simulink model "test_loadcase_moduleAssy_harness"  (R2026a)
settings: Solver=VariableStepAuto  StopTime=2000  AbsTol=1e-3
libraries: cooling_system_components x9, fl_lib x3, simulink x2, nesl_utility x2, pack_5p48s8p_detailled_Thr_library x1, pack_5p48s8p_1g10g1_Thr_library x1, pack_5p48s8p_1g10g1_5g1g5_Thr_library x1, pack_5p48s8p_Thr_library x1
Description:
  | Copyright 2023-2026 The MathWorks, Inc.
settings Model: Creator=smiller  LastModifiedBy=smiller
settings DebuggingCC: SymbolicDimsDataTypeCodeGenerationDiagnostic=none
settings SimscapeCC: SimscapeNominalValues="[{\"value\":\"1\",\"unit\":\"A\"},{\"value\":\"1\",\"unit\":\"bar\"},{\"value\":\"1\",\"unit\":\"cm^2\"},{\"value\":\"1\",\"unit\":\"cm^3/s\"},{\"value\":\"1\",\"unit\":\"kJ/kg\"},{\"value\":\"1\",\"unit\":\"kW\"},{\"value\":\"1\",\"unit\":\"l\"},{\"value\":\"1\",\"unit\":\"N\"},{\"value\":\"1\",\"unit\":\"N*m\"},{\"value\":\"1\",\"unit\":\"V\"}]"  SimscapeLogSimulationStatistics=on  SimscapeLogName=simlog_test_loadcase_module

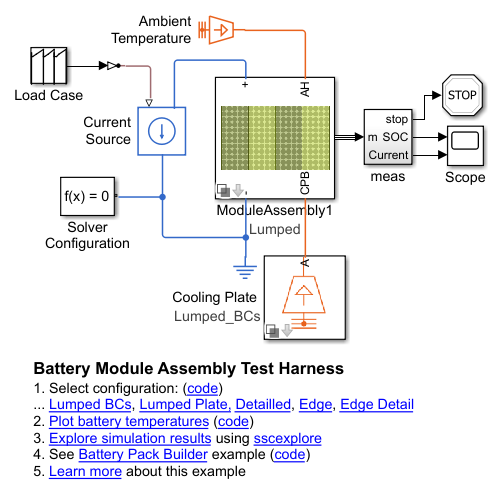
[thumbnail: Simulink's stored preview of the top-level diagram]
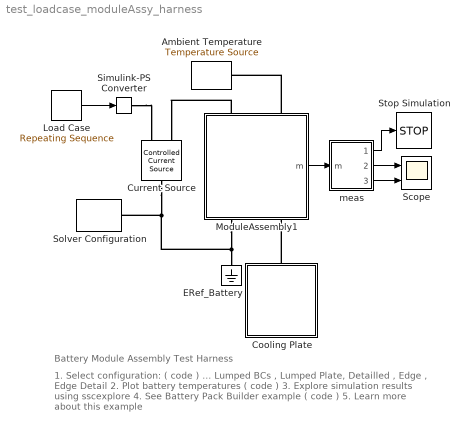
== system test_loadcase_moduleAssy_harness ==
  note: 1. Select configuration: ( code )
      | ... Lumped BCs , Lumped Plate, Detailled , Edge , Edge Detail
      | 2. Plot battery temperatures ( code )
      | 3. Explore simulation results using sscexplore
      | 4. See Battery Pack Builder example ( code )
      | 5. Learn more about this example
  note: Battery Module Assembly Test Harness
  Ambient Temperature : fl_lib/Thermal/Thermal Sources/Temperature Source  temperature=298 K
  Cooling Plate : Subsystem  Variant=on  VariantControlMode=label  VariantControl=Lumped_BCs  LabelModeActiveChoice=Lumped_BCs
      settings: AttributesFormatString=%<LabelModeActiveChoice>
  Current Source : fl_lib/Electrical/Electrical Sources/Controlled Current Source
  ERef_Battery : fl_lib/Electrical/Electrical Elements/Electrical Reference
  Load Case : simulink/Sources/Repeating Sequence  rep_seq_t="[0 1   2    32  33 300 800 2000]"  rep_seq_y=[0 0 450 450 400 400 440 510]/8
  ModuleAssembly1 : Subsystem  Variant=on  VariantControlMode=label  VariantControl=Choice  LabelModeActiveChoice=Lumped
      settings: AttributesFormatString=%<LabelModeActiveChoice>  PortSchema="{\"entries\":[{\"content\":{\"sides\":[{\"content\":{\"connectorIds\":[\"LConn1\",\"LConn2\"]},\"type\":\"ConnectorPlacement.EquallySpacedRectSide\",\"uuid\":\"bc91a472-35c0-4041-89a6-b649b08794f0\"},{\"content\":{\"connectorIds\":[\"RConn1\",\"RConn2\"],\"side\":\"RIGHT\"},\"type\":\"ConnectorPlacement.EquallySpacedRectSide\",\"uuid\":\"4a390b53-12a2-4d2f-9537-abc76db307f8\"},{\"content\":{\"connectorIds\":[],\"side\":\"TOP\"},\"type\":\"ConnectorPlacement.EquallySpacedRectSide\",\"uuid\":\"1a7ed896-4ada-4d88-995c-c24bd39ee86b\"},{\"content\":{\"connectorIds\":[\"Out1\"],\"side\":\"BOTTOM\"},\"type\":\"ConnectorPlacement.EquallySpacedRectSide\",\"uuid\":\"e36c911b-adc9-44cf-bfab-32777b2ec35c\"}]},\"type\":\"ConnectorPlacement.EquallySpacedConnector\",\"uuid\":\"4e67d65b-f12d-4d00-91b0-7eadb0a42625\"}],\"packageUris\":[\"http://schema.mathworks.com/mf0/Connector/R2020b\"],\"version\":\"1.0\"}"
  Scope : Scope  NumInputPorts=2
      settings: Title=Battery SOC  ActiveDisplayYMinimum=0.2125000000000116  ActiveDisplayYMaximum=1.0874999999999988
  Simulink-PS Converter : nesl_utility/Simulink-PS Converter  PhysicalDomain=network_engine_domain  SubClassName=ps_input  LeftPortType=input  RightPortType=output  PseudoPeriodic=off  Frequencies=[]  NoiseDistribution=none  NoiseParameters=[]  Unit=1  AffineConversion=off  FilteringAndDerivatives=filter  SimscapeFilterOrder=1  InputFilterTimeConstant=0.01  UdotUserProvided=0
  Solver Configuration : nesl_utility/Solver Configuration  PhysicalDomain=network_engine_domain  SubClassName=solver  LeftPortType=input  RightPortType=generic  Tones=[]  Harmonics=[]  SimulateNoise=off  Profile=off  UseLocalSampling=off  EnableSwitchedLinearOptims=on  FrequencyDomain=off  UseCCode=off  RelTol=0.001  AbsTol=1e-06  MinStep=1e-09  ToWorkspace=off  RevertToSquareIcSolve=off  NumHomotopyIterations=100  PhasorMode=off  PhasorModeNumHarmonics=1  ConsistencySolver=NEWTON_XTOL_AFTER_FTOL  CanonicalOrdering=UNORDERED  OptimizeIntermediates=UNOPTIMIZED  IndexReductionMethod=None  DoDC=off  ResidualTolerance=1e-09  ConsistencyTolSource=GLOBAL  ConsistencyAbsTol=0.001  ConsistencyRelTol=0.001  ConsistencyTolFactor=0.001  UseLocalSolver=off  LocalSolverChoice=NE_BACKWARD_EULER_ADVANCER  ResolveIndetEquations=on  FunctionEvalNumThread=1  LocalSolverSampleTime=0.001  DoFixedCost=off  MaxNonlinIter=3  MaxModeIter=2  ComputeImpulses=off  ImpulseIterations=2  LinearAlgebra=auto  LinearAlgebraNumThread=0  EquationFormulation=NE_TIME_EF  DelaysMemoryBudget=1024  AutomaticFiltering=on  FilteringTimeConstant=0.001  PartitionStorageMethod=AS_NEEDED  PartitionMemoryBudget=1024  PartitionMethod=ROBUST  MultibodyUseLocalSolver=off  MultibodyLocalSolverChoice=ODE1  MultibodyLocalSolverSampleTime=0.001
  Stop Simulation : Stop
  meas : Subsystem
  wires:
  Load Case/1 -> Simulink-PS Converter/1
  ModuleAssembly1/1(m) -> meas/1(m)
  meas/1(stop) -> Stop Simulation/1
  meas/2(SOC) -> Scope/1
  meas/3(Current) -> Scope/2
  connections:
  Solver Configuration/RConn1 -- ModuleAssembly1/RConn1 -- ERef_Battery/LConn1 -- Current Source/LConn1
  Simulink-PS Converter/RConn1 -- Current Source/RConn1
  ModuleAssembly1/LConn1 -- Current Source/RConn2
  ModuleAssembly1/LConn2 -- Ambient Temperature/LConn1
  Cooling Plate/LConn1 -- ModuleAssembly1/RConn2

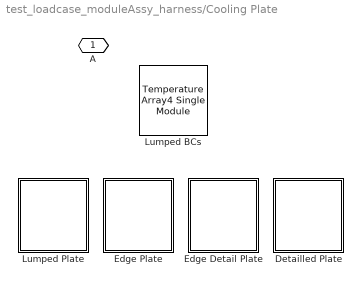
== system test_loadcase_moduleAssy_harness/Cooling Plate ==
  Detailled Plate : Subsystem  VariantControl=Detailled_Plate
      mask Display: image('ssc_airvtol_cooling_plate_IMAGE.png');
  Edge Plate : Subsystem  VariantControl=Edge_Plate
      mask Display: image('ssc_airvtol_cooling_plate_IMAGE.png');
  Edge Detail Plate : Subsystem  VariantControl=Edge_Detail_Plate
      mask Display: image('ssc_airvtol_cooling_plate_IMAGE.png');
  Lumped BCs : cooling_system_components/Temperature Array4 Single Module  VariantControl=Lumped_BCs  t_in=23  t_out=26
  Lumped Plate : Subsystem  VariantControl=Lumped_Plate
      mask Display: image('ssc_airvtol_cooling_plate_IMAGE.png');
  A : PMIOPort  Side=Left

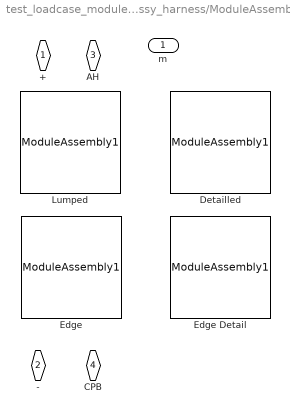
== system test_loadcase_moduleAssy_harness/ModuleAssembly1 ==
  Detailled : pack_5p48s8p_detailled_Thr_library/ModuleAssembly1  VariantControl=Detailled  Cell=ModuleType1_det  Targets=targets_5p48s8p_detailled_thr.ModuleAssembly1  BatteryObj=batt_5p12s_detailled_thr
  Edge : pack_5p48s8p_1g10g1_Thr_library/ModuleAssembly1  VariantControl=Edge  Cell=ModuleType1  Targets=targets_5p48s8p_1g10g1_thr.ModuleAssembly1  BatteryObj=batt_5p48s_1g10g1_thr
  Edge Detail : pack_5p48s8p_1g10g1_5g1g5_Thr_library/ModuleAssembly1  VariantControl=Edge_Detail  Cell=ModuleType1  Targets=targets_5p48s8p_1g10g1_5g1g5_thr.ModuleAssembly1  BatteryObj=batt_5p48s_1g10g1_5g1g5_thr
  Lumped : pack_5p48s8p_Thr_library/ModuleAssembly1  VariantControl=Lumped  Cell=ModuleType1  Targets=targets_5p48s8p_thr.ModuleAssembly1  BatteryObj=batt_5p48s_thr
  + : PMIOPort  Side=Left
  - : PMIOPort  Port=2  Side=Right
  AH : PMIOPort  Port=3  Side=Left
  CPB : PMIOPort  Port=4  Side=Right
  m : Outport

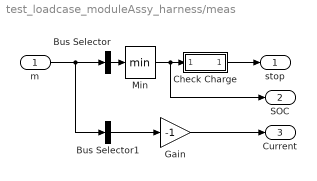
== system test_loadcase_moduleAssy_harness/meas ==
  m : Inport
  Bus Selector : BusSelector  OutputSignals=socC.M1  OutputAsBus=on
  Bus Selector1 : BusSelector  OutputSignals=i.M1  OutputAsBus=on
  Check Charge : Subsystem  mask{q_battery_limit=0.3}
      mask prompts: q_battery_limit "Battery charge lower limit (A*hr)"
  Gain : Gain  Gain=-1
  Min : MinMax
  stop : Outport
  SOC : Outport  Port=2
  Current : Outport  Port=3
  wires:
  Min/1 -> SOC/1, Check Charge/1(In1)
  m/1 -> Bus Selector1/1, Bus Selector/1
  Bus Selector1/1 -> Gain/1
  Bus Selector/1 -> Min/1
  Check Charge/1(stop) -> stop/1
  Gain/1 -> Current/1

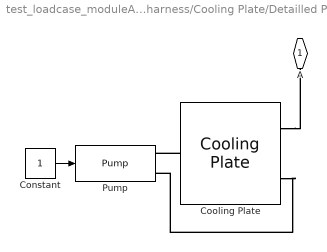
== system test_loadcase_moduleAssy_harness/Cooling Plate/Detailled Plate ==
  Constant : Constant
  Cooling Plate : cooling_system_components/Cooling Plate  plate=plate_5p48s_detailled_thr
  Pump : cooling_system_components/Pump  num_plates=1
  A : PMIOPort  Side=Left
  wires:
  Constant/1 -> Pump/1
  connections:
  Cooling Plate/LConn2 -- Pump/RConn2
  Cooling Plate/RConn1 -- Pump/RConn1
  Cooling Plate/LConn1 -- A/RConn1

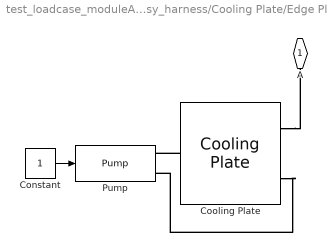
== system test_loadcase_moduleAssy_harness/Cooling Plate/Edge Plate ==
  Constant : Constant
  Cooling Plate : cooling_system_components/Cooling Plate  plate=plate_5p48s_1g10g1_thr
  Pump : cooling_system_components/Pump  num_plates=1
  A : PMIOPort  Side=Left
  wires:
  Constant/1 -> Pump/1
  connections:
  Cooling Plate/LConn2 -- Pump/RConn2
  Cooling Plate/RConn1 -- Pump/RConn1
  Cooling Plate/LConn1 -- A/RConn1

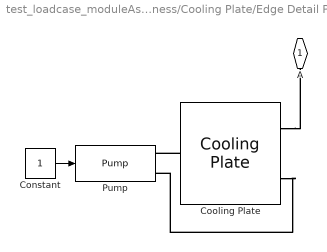
== system test_loadcase_moduleAssy_harness/Cooling Plate/Edge Detail Plate ==
  Constant : Constant
  Cooling Plate : cooling_system_components/Cooling Plate  plate=plate_5p48s_1g10g1_5g1g5_thr
  Pump : cooling_system_components/Pump  num_plates=1
  A : PMIOPort  Side=Left
  wires:
  Constant/1 -> Pump/1
  connections:
  Cooling Plate/LConn1 -- A/RConn1
  Cooling Plate/RConn1 -- Pump/RConn1
  Cooling Plate/LConn2 -- Pump/RConn2

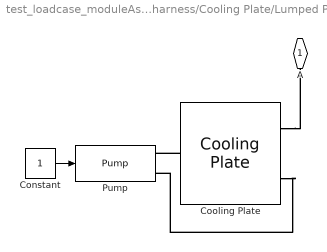
== system test_loadcase_moduleAssy_harness/Cooling Plate/Lumped Plate ==
  Constant : Constant
  Cooling Plate : cooling_system_components/Cooling Plate  plate=plate_5p48s_thr
  Pump : cooling_system_components/Pump  num_plates=1
  A : PMIOPort  Side=Left
  wires:
  Constant/1 -> Pump/1
  connections:
  Cooling Plate/LConn1 -- A/RConn1
  Cooling Plate/RConn1 -- Pump/RConn1
  Cooling Plate/LConn2 -- Pump/RConn2

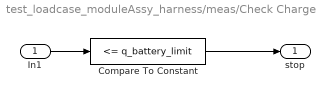
== system test_loadcase_moduleAssy_harness/meas/Check Charge ==
  In1 : Inport
  Compare To Constant : simulink/Logic and Bit Operations/Compare To Constant  relop=<=  const=q_battery_limit  OutDataTypeStr=boolean
  stop : Outport  VectorParamsAs1DForOutWhenUnconnected=off
  wires:
  Compare To Constant/1 -> stop/1
  In1/1 -> Compare To Constant/1
